simulink model "DrivingDistance"  (R2018b)
settings: Solver=VariableStepAuto  StartTime=0.0  StopTime=1000  RelTol=1e-3
settings Model: Creator=gregoryseibert  LastModifiedBy=gregoryseibert

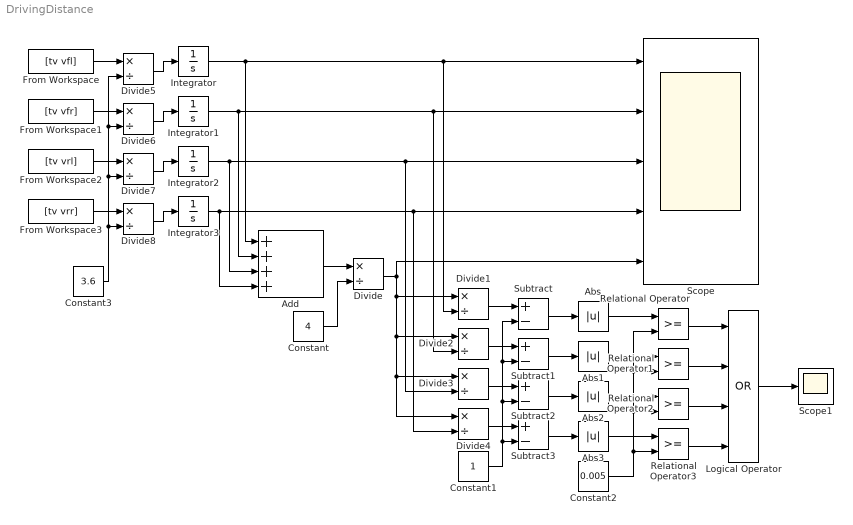
== system DrivingDistance ==
  Abs{,1..3} (4 alike) : Abs
  Add : Sum  Inputs=++++
  Constant : Constant  Value=4
  Constant1 : Constant
  Constant2 : Constant  Value=0.005
  Constant3 : Constant  Value=3.6
  Divide{,1..8} (9 alike) : Product  Inputs=*/
  From Workspace : FromWorkspace  VariableName=[tv vfl]  SampleTime=0
  From Workspace1 : FromWorkspace  VariableName=[tv vfr]  SampleTime=0
  From Workspace2 : FromWorkspace  VariableName=[tv vrl]  SampleTime=0
  From Workspace3 : FromWorkspace  VariableName=[tv vrr]  SampleTime=0
  Integrator{,1..3} (4 alike) : Integrator
  Logical Operator : Logic  Operator=OR  Inputs=4  AllPortsSameDT=off  OutDataTypeStr=boolean
  Relational Operator{,1..3} (4 alike) : RelationalOperator  OutDataTypeStr=boolean  RndMeth=Simplest
  Scope : Scope  NumInputPorts=5
  Scope1 : Scope
  Subtract{,1..3} (4 alike) : Sum  Inputs=+-
  wires:
  Integrator/1 -> Divide1/2, Scope/1, Add/1
  Integrator1/1 -> Divide2/2, Scope/2, Add/2
  Integrator2/1 -> Scope/3, Divide3/2, Add/3
  Integrator3/1 -> Divide4/2, Scope/4, Add/4
  Add/1 -> Divide/1
  Constant/1 -> Divide/2
  Divide/1 -> Divide4/1, Divide3/1, Divide2/1, Divide1/1, Scope/5
  Divide1/1 -> Subtract/1
  Divide2/1 -> Subtract1/1
  Divide3/1 -> Subtract2/1
  Divide4/1 -> Subtract3/1
  Constant1/1 -> Subtract3/2, Subtract2/2, Subtract/2, Subtract1/2
  Subtract1/1 -> Abs1/1
  Subtract/1 -> Abs/1
  Subtract2/1 -> Abs2/1
  Subtract3/1 -> Abs3/1
  Abs/1 -> Relational Operator/1
  Abs1/1 -> Relational Operator1/1
  Abs2/1 -> Relational Operator2/1
  Abs3/1 -> Relational Operator3/1
  Logical Operator/1 -> Scope1/1
  Relational Operator/1 -> Logical Operator/1
  Relational Operator1/1 -> Logical Operator/2
  Relational Operator2/1 -> Logical Operator/3
  Relational Operator3/1 -> Logical Operator/4
  Constant2/1 -> Relational Operator/2, Relational Operator1/2, Relational Operator2/2, Relational Operator3/2
  From Workspace1/1 -> Divide6/1
  From Workspace2/1 -> Divide7/1
  From Workspace3/1 -> Divide8/1
  Divide5/1 -> Integrator/1
  From Workspace/1 -> Divide5/1
  Divide8/1 -> Integrator3/1
  Divide7/1 -> Integrator2/1
  Divide6/1 -> Integrator1/1
  Constant3/1 -> Divide5/2, Divide6/2, Divide7/2, Divide8/2
